simulink model "SimulinkPrimerArmonicoMuestreoR2018a"  (R2018a)
settings: Solver=ode5  StartTime=0.0  StopTime=1  FixedStep=0.01  RelTol=1e-3
settings Model: Creator=aghersin  LastModifiedBy=aghersin
settings CodeAppCC: StateflowObjectComments=on

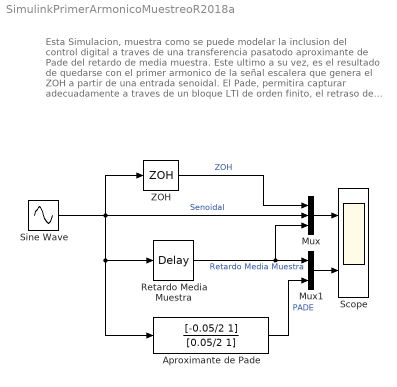
== system SimulinkPrimerArmonicoMuestreoR2018a ==
  note: Esta Simulacion, muestra como se puede modelar la inclusion del
      | control digital a traves de una transferencia pasatodo aproximante
      | de Pade del retardo de media muestra. Este ultimo a su vez, es el
      | resultado de quedarse con el primer armonico de la señal escalera
      | que genera el ZOH a partir de una entrada senoidal. El Pade,
      | permitira capturar adecuadamente a traves de un bloque LTI de
      | orden finito, el retraso de fase introducido por el control digital.
      | Muestreo: .1 seg.
  Aproximante de Pade : TransferFcn  Numerator=[-0.05/2 1]  Denominator=[0.05/2 1]
  Mux : Mux  Inputs=3
  Mux1 : Mux  Inputs=2
  Retardo Media Muestra : TransportDelay  DelayTime=.05
  Scope : Scope  NumInputPorts=2
  Sine Wave : Sin  Frequency=2*pi  SampleTime=0
  ZOH : ZeroOrderHold  SampleTime=.1
  wires:
  Aproximante de Pade/1 -> Mux1/2  "PADE"
  ZOH/1 -> Mux/1  "ZOH"
  Mux1/1 -> Scope/2
  Sine Wave/1 -> Retardo Media Muestra/1, Aproximante de Pade/1, Mux/2, ZOH/1  "Senoidal"
  Mux/1 -> Scope/1
  Retardo Media Muestra/1 -> Mux/3, Mux1/1  "Retardo Media Muestra"
